simulink model "feedforwardOptimizer"  (R2019a)
settings: Solver=ode2  StartTime=0.0  StopTime=300  FixedStep=0.1  RelTol=1e-3
settings Model: Creator=HP  LastModifiedBy=swastik
settings DataIOCC: ReturnWorkspaceOutputs=off
settings DebuggingCC: ArithmeticOperatorsInVariantConditions=warning

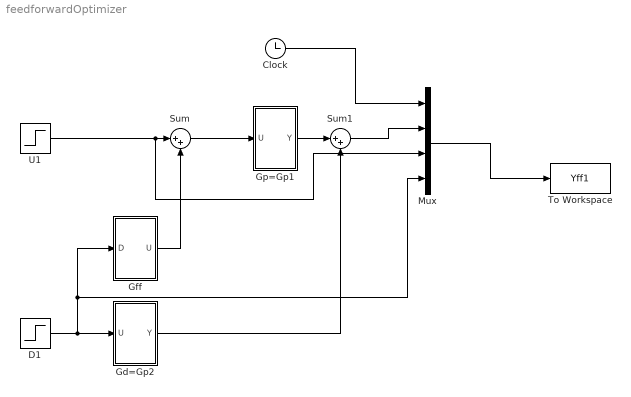
== system feedforwardOptimizer ==
  Clock : Clock
  D1 : Step  Time=0  SampleTime=0
  Gd=Gp2 : Subsystem  mask{K2=0.9894, T2=26.1, D2=20.6}
      mask prompts: K2 "Gain"; T2 "Lag time"; D2 "Dead Time"
  Gff : Subsystem  mask{Tp=15.436, Td=24.445, D=6.1507}
      mask prompts: Tp "Lead"; Td "Lag"; D "Dead time"
  Gp=Gp1 : Subsystem  mask{K=1.9886, T=17.4, D=14}
      mask prompts: K "Gain"; T "Lag Time"; D "Dead Time"
  Mux : Mux
  Sum : Sum  Inputs=|++
  Sum1 : Sum  Inputs=|++
  To Workspace : ToWorkspace  VariableName=Yff1  SampleTime=-1
  U1 : Step  Time=0  After=0  SampleTime=0
  wires:
  Clock/1 -> Mux/1
  Mux/1 -> To Workspace/1
  D1/1 -> Gd=Gp2/1(U), Gff/1(D), Mux/4
  U1/1 -> Mux/3, Sum/1
  Gff/1(U) -> Sum/2
  Sum/1 -> Gp=Gp1/1(U)
  Gp=Gp1/1(Y) -> Sum1/1
  Gd=Gp2/1(Y) -> Sum1/2
  Sum1/1 -> Mux/2

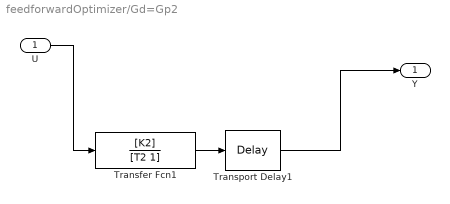
== system feedforwardOptimizer/Gd=Gp2 ==
  U : Inport
  Transfer Fcn1 : TransferFcn  Numerator=[K2]  Denominator=[T2 1]
  Transport Delay1 : TransportDelay  DelayTime=D2
  Y : Outport
  wires:
  Transfer Fcn1/1 -> Transport Delay1/1
  Transport Delay1/1 -> Y/1
  U/1 -> Transfer Fcn1/1

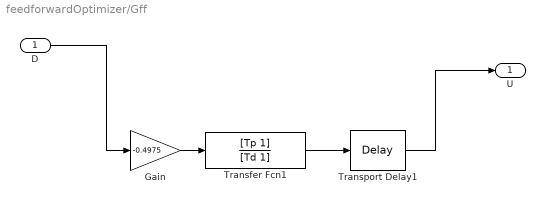
== system feedforwardOptimizer/Gff ==
  D : Inport
  Gain : Gain  Gain=-0.4975
  Transfer Fcn1 : TransferFcn  Numerator=[Tp 1]  Denominator=[Td 1]
  Transport Delay1 : TransportDelay  DelayTime=D
  U : Outport
  wires:
  Transfer Fcn1/1 -> Transport Delay1/1
  Transport Delay1/1 -> U/1
  Gain/1 -> Transfer Fcn1/1
  D/1 -> Gain/1

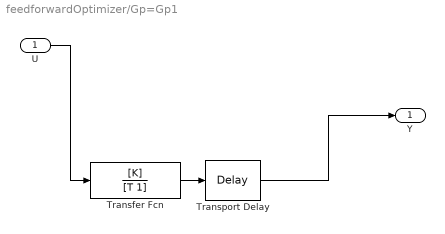
== system feedforwardOptimizer/Gp=Gp1 ==
  U : Inport
  Transfer Fcn : TransferFcn  Numerator=[K]  Denominator=[T 1]
  Transport Delay : TransportDelay  DelayTime=D
  Y : Outport
  wires:
  Transfer Fcn/1 -> Transport Delay/1
  U/1 -> Transfer Fcn/1
  Transport Delay/1 -> Y/1
